simulink model "nouveaux_graphes1"  (R2018a)
settings: Solver=VariableStepAuto  StartTime=0.0  StopTime=1000  RelTol=1e-3
libraries: simulink x2
settings Model: Creator=ITEC  LastModifiedBy=ITEC

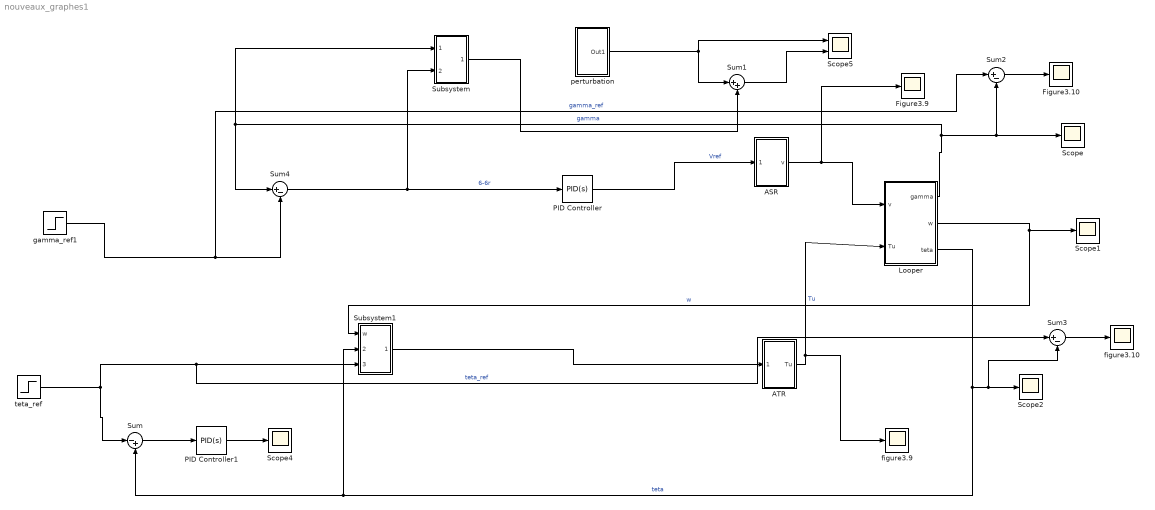
== system nouveaux_graphes1 ==
  ASR : Subsystem
  ATR : Subsystem
  Figure3.10 : Scope
  Figure3.9 : Scope
  Looper : Subsystem
  PID Controller : simulink/Continuous/PID Controller  Controller=PID  TimeDomain=Continuous-time  SampleTime=-1  IntegratorMethod=Forward Euler  FilterMethod=Forward Euler  Form=Parallel  UseFilter=on  ControllerParametersSource=internal  P=2.23508121014437e-11  I=1.06368013737669e-12  D=1.00402084111458e-10  N=1.09110813516919  InitialConditionSource=internal  InitialConditionForIntegrator=0  InitialConditionForFilter=0  ExternalReset=none  LimitOutput=off  UpperSaturationLimit=inf  LowerSaturationLimit=-inf  LinearizeAsGain=on  AntiWindupMode=none  Kb=1  TrackingMode=off  Kt=1  PParamMin=[]  PParamMax=[]  IParamMin=[]  IParamMax=[]  DParamMin=[]  DParamMax=[]  NParamMin=[]  NParamMax=[]  KbParamMin=[]  KbParamMax=[]  KtParamMin=[]  KtParamMax=[]  POutMin=[]  POutMax=[]  IOutMin=[]  IOutMax=[]  DOutMin=[]  DOutMax=[]  NOutMin=[]  NOutMax=[]  KbOutMin=[]  KbOutMax=[]  KtOutMin=[]  KtOutMax=[]  IntegratorOutMin=[]  IntegratorOutMax=[]  FilterOutMin=[]  FilterOutMax=[]  SumOutMin=[]  SumOutMax=[]  SumI1OutMin=[]  SumI1OutMax=[]  SumI2OutMin=[]  SumI2OutMax=[]  SumI3OutMin=[]  SumI3OutMax=[]  SumDOutMin=[]  SumDOutMax=[]  SaturationOutMin=[]  SaturationOutMax=[]  IntegratorContinuousStateAttributes=''  IntegratorStateMustResolveToSignalObject=off  IntegratorRTWStateStorageClass=Auto  FilterContinuousStateAttributes=''  FilterStateMustResolveToSignalObject=off  FilterRTWStateStorageClass=Auto  DifferentiatorICPrevScaledInput=0  DifferentiatorOutMin=[]  DifferentiatorOutMax=[]  FilterDiffOutCoefMin=[]  FilterDiffOutCoefMax=[]  SumDenOutMin=[]  SumDenOutMax=[]  SumNumOutMin=[]  SumNumOutMax=[]  ReciprocalOutMin=[]  ReciprocalOutMax=[]  DivideOutMin=[]  DivideOutMax=[]  TunerSelectOption=Transfer Function Based (PID Tuner App)
  PID Controller1 : simulink/Continuous/PID Controller  Controller=PID  TimeDomain=Continuous-time  SampleTime=-1  IntegratorMethod=Forward Euler  FilterMethod=Forward Euler  Form=Parallel  UseFilter=on  ControllerParametersSource=internal  P=-296.60353357804  I=-0.16042431692249  D=-102333.934744472  N=0.0218878390511582  InitialConditionSource=internal  InitialConditionForIntegrator=0  InitialConditionForFilter=0  ExternalReset=none  LimitOutput=off  UpperSaturationLimit=inf  LowerSaturationLimit=-inf  LinearizeAsGain=on  AntiWindupMode=none  Kb=1  TrackingMode=off  Kt=1  PParamMin=[]  PParamMax=[]  IParamMin=[]  IParamMax=[]  DParamMin=[]  DParamMax=[]  NParamMin=[]  NParamMax=[]  KbParamMin=[]  KbParamMax=[]  KtParamMin=[]  KtParamMax=[]  POutMin=[]  POutMax=[]  IOutMin=[]  IOutMax=[]  DOutMin=[]  DOutMax=[]  NOutMin=[]  NOutMax=[]  KbOutMin=[]  KbOutMax=[]  KtOutMin=[]  KtOutMax=[]  IntegratorOutMin=[]  IntegratorOutMax=[]  FilterOutMin=[]  FilterOutMax=[]  SumOutMin=[]  SumOutMax=[]  SumI1OutMin=[]  SumI1OutMax=[]  SumI2OutMin=[]  SumI2OutMax=[]  SumI3OutMin=[]  SumI3OutMax=[]  SumDOutMin=[]  SumDOutMax=[]  SaturationOutMin=[]  SaturationOutMax=[]  IntegratorContinuousStateAttributes=''  IntegratorStateMustResolveToSignalObject=off  IntegratorRTWStateStorageClass=Auto  FilterContinuousStateAttributes=''  FilterStateMustResolveToSignalObject=off  FilterRTWStateStorageClass=Auto  DifferentiatorICPrevScaledInput=0  DifferentiatorOutMin=[]  DifferentiatorOutMax=[]  FilterDiffOutCoefMin=[]  FilterDiffOutCoefMax=[]  SumDenOutMin=[]  SumDenOutMax=[]  SumNumOutMin=[]  SumNumOutMax=[]  ReciprocalOutMin=[]  ReciprocalOutMax=[]  DivideOutMin=[]  DivideOutMax=[]  TunerSelectOption=Transfer Function Based (PID Tuner App)
  Scope{,1..2,4} (4 alike) : Scope
  Scope5 : Scope  NumInputPorts=2
  Subsystem : Subsystem
  Subsystem1 : Subsystem
  Sum : Sum  Inputs=|-+
  Sum1 : Sum  Inputs=|++
  Sum2 : Sum  Inputs=|+-
  Sum3 : Sum  Inputs=|+-
  Sum4 : Sum  Inputs=|+-
  figure3.10 : Scope
  figure3.9 : Scope
  gamma_ref1 : Step  Time=100  After=8*(10e6)  SampleTime=0
  perturbation : Subsystem
  teta_ref : Step  Time=100  After=0.3491  SampleTime=0
  wires:
  Sum/1 -> PID Controller1/1
  ATR/1(Tu) -> figure3.9/1, Looper/2(Tu)  "Tu"
  perturbation/1(Out1) -> Sum1/1, Scope5/1
  Looper/3(teta) -> Sum3/2, Scope2/1, Sum/2, Subsystem1/2(teta)  "teta"
  Sum1/1 -> Scope5/2
  Subsystem/1(Vref) -> Sum1/2
  Looper/1(gamma) -> Subsystem/1(gamma), Sum4/1, Sum2/2, Scope/1  "gamma"
  Looper/2(w) -> Subsystem1/1(w), Scope1/1  "w"
  Sum4/1 -> Subsystem/2(6-6r), PID Controller/1  "6-6r"
  teta_ref/1 -> Sum/1, Sum3/1, Subsystem1/3(teta_ref)  "teta_ref"
  gamma_ref1/1 -> Sum2/1, Sum4/2  "gamma_ref"
  PID Controller1/1 -> Scope4/1
  ASR/1(v) -> Figure3.9/1, Looper/1(v)
  PID Controller/1 -> ASR/1(Vref)  "Vref"
  Subsystem1/1(Turef) -> ATR/1(Turef)
  Sum2/1 -> Figure3.10/1
  Sum3/1 -> figure3.10/1

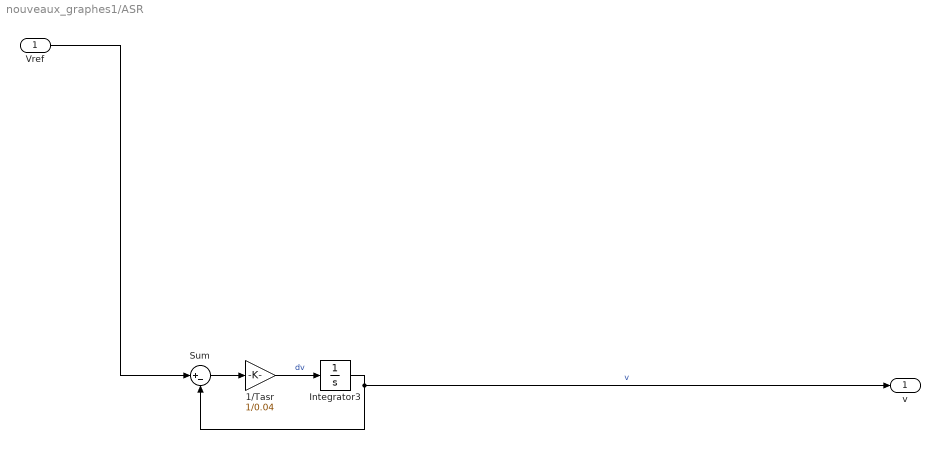
== system nouveaux_graphes1/ASR ==
  Vref : Inport
  1/Tasr : Gain  Gain=1/0.04
  Integrator3 : Integrator
  Sum : Sum  Inputs=|+-
  v : Outport
  wires:
  Sum/1 -> 1/Tasr/1
  Vref/1 -> Sum/1
  1/Tasr/1 -> Integrator3/1  "dv"
  Integrator3/1 -> v/1, Sum/2  "v"

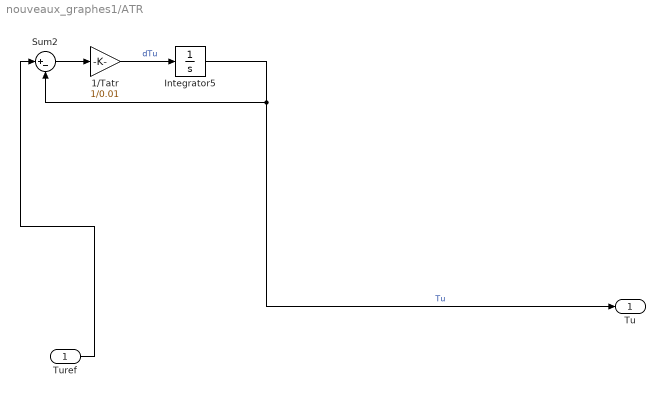
== system nouveaux_graphes1/ATR ==
  Turef : Inport
  1/Tatr : Gain  Gain=1/0.01
  Integrator5 : Integrator
  Sum2 : Sum  Inputs=|+-
  Tu : Outport
  wires:
  Integrator5/1 -> Tu/1, Sum2/2  "Tu"
  1/Tatr/1 -> Integrator5/1  "dTu"
  Sum2/1 -> 1/Tatr/1
  Turef/1 -> Sum2/1

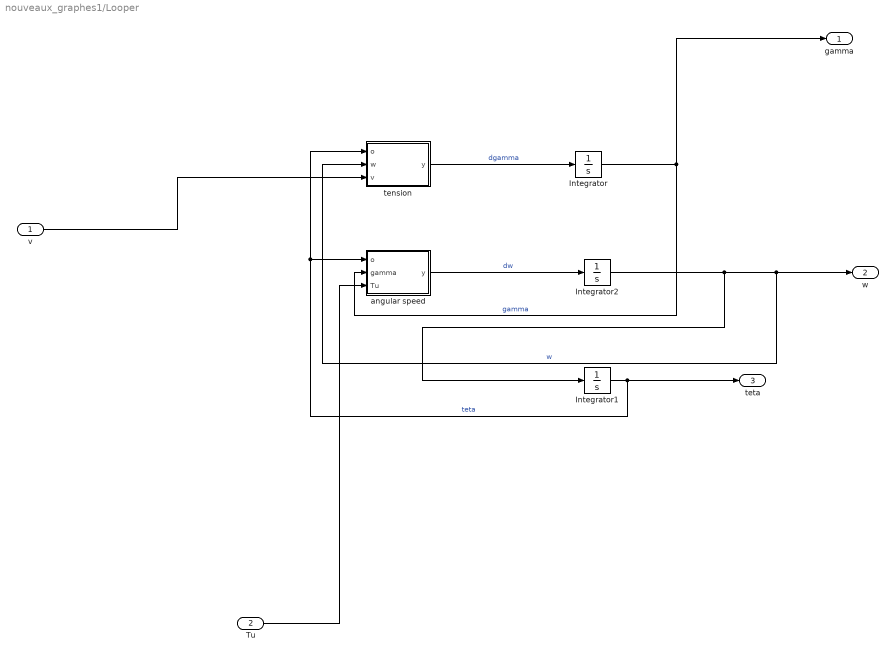
== system nouveaux_graphes1/Looper ==
  v : Inport
  Tu : Inport  Port=2
  Integrator : Integrator
  Integrator1 : Integrator
  Integrator2 : Integrator
  angular speed : MATLAB Function  TreatAsAtomicUnit=on
  tension : MATLAB Function  TreatAsAtomicUnit=on
  gamma : Outport
  w : Outport  Port=2
  teta : Outport  Port=3
  wires:
  Tu/1 -> angular speed/3(Tu)
  Integrator2/1 -> w/1, tension/2(w), Integrator1/1  "w"
  tension/1(y) -> Integrator/1  "dgamma"
  Integrator/1 -> gamma/1, angular speed/2(gamma)  "gamma"
  angular speed/1(y) -> Integrator2/1  "dw"
  Integrator1/1 -> teta/1, tension/1(o), angular speed/1(o)  "teta"
  v/1 -> tension/3(v)

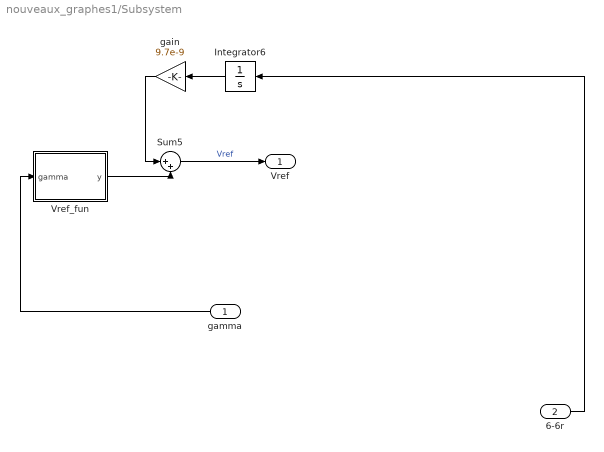
== system nouveaux_graphes1/Subsystem ==
  gamma : Inport
  6-6r : Inport  Port=2
  Integrator6 : Integrator
  Sum5 : Sum  Inputs=|++
  Vref_fun : MATLAB Function  TreatAsAtomicUnit=on
  gain : Gain  Gain=9.7e-9
  Vref : Outport
  wires:
  Sum5/1 -> Vref/1  "Vref"
  Integrator6/1 -> gain/1
  gamma/1 -> Vref_fun/1(gamma)
  gain/1 -> Sum5/1
  6-6r/1 -> Integrator6/1
  Vref_fun/1(y) -> Sum5/2

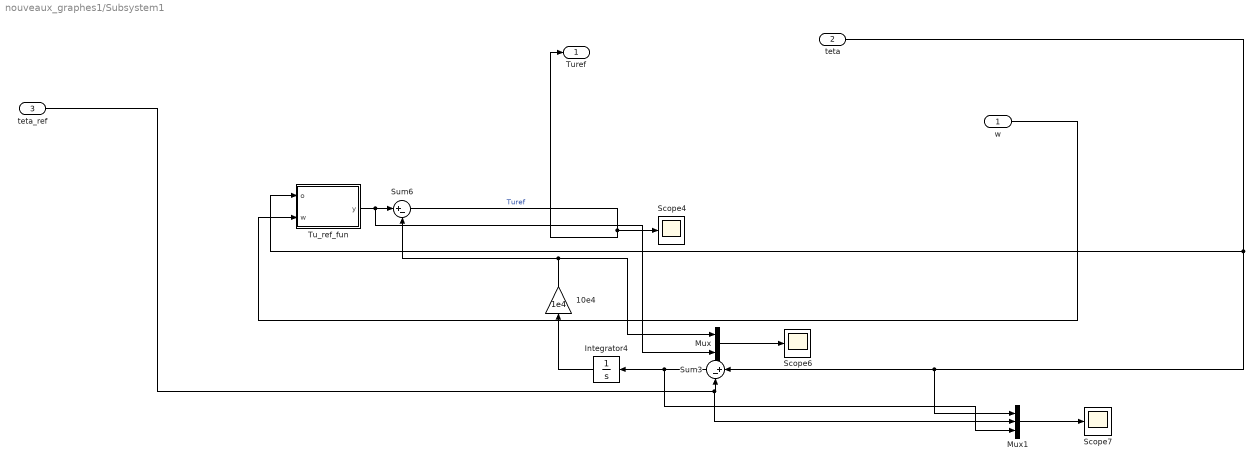
== system nouveaux_graphes1/Subsystem1 ==
  w : Inport
  teta : Inport  Port=2
  teta_ref : Inport  Port=3
  10e4 : Gain  Gain=1e4
  Integrator4 : Integrator
  Mux : Mux  Inputs=2
  Mux1 : Mux  Inputs=3
  Scope4 : Scope
  Scope6 : Scope
  Scope7 : Scope
  Sum3 : Sum  Inputs=|+-
  Sum6 : Sum  Inputs=|+-
  Tu_ref_fun : MATLAB Function  TreatAsAtomicUnit=on
  Turef : Outport
  wires:
  Mux1/1 -> Scope7/1
  teta/1 -> Mux1/1, Sum3/1, Tu_ref_fun/1(o)
  Sum6/1 -> Turef/1, Scope4/1  "Turef"
  10e4/1 -> Sum6/2, Mux/1
  Tu_ref_fun/1(y) -> Mux/2, Sum6/1
  Mux/1 -> Scope6/1
  w/1 -> Tu_ref_fun/2(w)
  teta_ref/1 -> Mux1/2, Sum3/2
  Sum3/1 -> Integrator4/1, Mux1/3
  Integrator4/1 -> 10e4/1

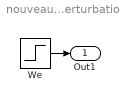
== system nouveaux_graphes1/perturbation ==
  We : Step  After=0.01  SampleTime=0
  Out1 : Outport
  wires:
  We/1 -> Out1/1

== matlab function nouveaux_graphes1/Subsystem1/Tu_ref_fun ==
  data: o input; y output; w input
function y = fcn(o,w)
Ro=7800;
h=0.00728;
wc=1.5;
Rl=0.611;
g=9.8;
Ml=1862.9;
Rg=0.194;
J=172.65;
L1=2.34;
Rr=0.0925;
L4=3.46;
H1=0.195;
E=1.2e10;
gamma_r=8e6;
o_r=0.3491;
Tu0=0;
Tu_ref= Tu0 -(8e3)*(o-o_r) - (7e3)*w
y = Tu_ref;

== matlab function nouveaux_graphes1/Subsystem/Vref_fun ==
  data: gamma input; y output
function y = fcn(gamma)
Ro=7800;
h=0.00728;
wc=1.5;
Rl=0.611;
g=9.8;
Ml=1862.9;
Rg=0.194;
J=172.65;
L1=2.34;
Rr=0.0925;
L4=3.46;
H1=0.195;
E=1.2e10;
gamma_r=8e6;
o_r=0.3491;
Tu0=0;
vref=(9.7e-10)*(gamma-gamma_r) ;
y = vref;

== matlab function nouveaux_graphes1/Looper/tension ==
  data: o input; y output; w input; v input
function y = fcn(o,w,v)
Ro=7800;
h=0.00728;
wc=1.5;
Rl=0.611;
g=9.8;
Ml=1862.9;
Rg=0.194;
J=172.65;
L1=2.34;
Rr=0.0925;
L4=3.46;
H1=0.195;
E=1.2e10;
gamma_r=8e6;
o_r=0.3491;
Tu0=0;
%L=sqrt((L1+Rl*cos(o))^(2)+(Rl*sin(o)+Rr-H1)^(2))+sqrt((L4+Rl*cos(o))^(2)+(Rl*sin(o)+Rr-H1)^(2));
L=5.8;
a=atan((Rl*sin(o)-H1+Rr)/(L1+Rl*cos(o)));
B=atan((Rl*sin(o)-H1+Rr)/(L4-Rl*cos(o)));
F3=Rl*(sin(o+B)-sin(o-a));
gamma_p=(E/L)*(F3*w-v);
y = gamma_p;

== matlab function nouveaux_graphes1/Looper/angular speed ==
  data: o input; y output; gamma input; Tu input
function y = fcn(o,gamma,Tu)
Ro=7800;
h=0.00728;
wc=1.5;
Rl=0.611;
g=9.8;
Ml=1862.9;
Rg=0.194;
J=172.65;
L1=2.34;
Rr=0.0925;
L4=3.46;
H1=0.195;
E=1.2e10;
gamma_r=8e6;
o_r=0.3491;
Tu0=0;
%L=sqrt((L1+Rl*cos(o))^(2)+(Rl*sin(o)+Rr-H1)^(2))+sqrt((L4+Rl*cos(o))^(2)+(Rl*sin(o)+Rr-H1)^(2))
L=5.8;
a=atan((Rl*sin(o)-H1+Rr)/(L1+Rl*cos(o)))
B=atan((Rl*sin(o)-H1+Rr)/(L4-Rl*cos(o)))
F1=0.5*g*Ro*L*h*wc*Rl*cos(o)+g*Ml*Rg*cos(o)
F3=Rl*(sin(o+B)-sin(o-a))
A=h*wc
w_p=(1/J)*(Tu-F1-gamma*A*F3)  %+Ww)
y = w_p;
